simulink model "pos_8mot"  (R2021a)
settings: Solver=FixedStepDiscrete  StartTime=0.0  StopTime=inf  FixedStep=0.001  RelTol=1e-3  EnableMultiTasking=on
InitFcn:
  | load("rho_CommandCalib.mat");
  | run("importCmd.m")
model workspace (MAT data in the model file):
  positionCmd = [145.742 145.741 145.741 145.74 145.74 145.739 145.738 145.738 145.737 145.737 145.736 145.735 ... (560000 elements, 70000x8)]
  tempsTraj = [25 25 20]
values from neighbouring files (symbols this model uses):
  rho_CommandCalib = [325.033 325.033 325.033 325.033 325.033 325.033 325.033 325.033 325.033 325.033 325.033 325.033 ... (80000 elements, 10000x8)]    [rho_CommandCalib.mat]
undefined symbols (not defined in the file or in its folder): rho_CommandCircXY, rho_CommandCroixTilt, rho_CommandCroixXY, rho_CommandInclinaison, rho_CommandInclinaisonInterieure, rho_CommandPickAndPlace, rho_CommandPickAndPlaceTilt, rho_CommandPickAndPlaceVertical, rho_CommandPickAndPlaceX, rho_CommandSinusZ, rho_CommandSinusZ_decentree, rho_CommandTwist
libraries: xpcethercatlib x64, slrealtimeethercatlib x36, commutil2 x19, slrealtimeobsoletelib x7
(part 1 of 3)
settings Model: xpc_rtwmakecfg_data=_xpcethercatlib_  SimulationMode=external  OrderedModelArguments=off  Creator=The MathWorks, Inc.  LastModifiedBy=MNLER
settings SolverCC: AlgebraicLoopSolver=TrustRegion
settings DataIOCC: LimitDataPoints=on  SaveFinalState=on  SaveFormat=StructureWithTime  InspectSignalLogs=on  ReturnWorkspaceOutputs=off
settings OptimizationCC: BlockReduction=off  OptimizeBlockIOStorage=off  BufferReuse=off  GlobalBufferReuse=off  ExpressionFolding=off  ExpressionDepthLimit=2147483647  LocalBlockOutputs=off  LifeSpan=inf  OptimizeDataStoreBuffers=off  BusAssignmentInplaceUpdate=off
settings DebuggingCC: RTPrefix=none  ReadBeforeWriteMsg=DisableAll  WriteAfterWriteMsg=DisableAll  WriteAfterReadMsg=DisableAll  UnderspecifiedInitializationDetection=Classic  MergeDetectMultiDrivingBlocksExec=none  MaxConsecutiveZCsMsg=warning  SolverPrmCheckMsg=warning  InheritedTsInSrcMsg=none  MultiTaskDSMMsg=none  MultiTaskCondExecSysMsg=none  MultiTaskRateTransMsg=warning  TasksWithSamePriorityMsg=none  SigSpecEnsureSampleTimeMsg=none  Int32ToFloatConvMsg=none  ParameterDowncastMsg=none  ParameterOverflowMsg=none  ParameterPrecisionLossMsg=none  ParameterTunabilityLossMsg=none  FcnCallInpInsideContextMsg=warning  BusObjectLabelMismatch=none  RootOutportRequireBusObject=none  ModelReferenceExtraNoncontSigs=none  StateNameClashWarn=warning  NonCurrentReleaseOperatingPointMsg=warning  SFUnexpectedBacktrackingDiag=warning  SFNoUnconditionalDefaultTransitionDiag=warning  SFExecutionAtInitializationDiag=none  SFMachineParentedDataDiag=warning  ArithmeticOperatorsInVariantConditions=warning
settings HardwareCC: ProdBitPerPointer=32  ProdBitPerSizeT=32  ProdBitPerPtrDiffT=32  ProdLargestAtomicFloat=None  ProdWordSize=32  ProdLongLongMode=on  ProdHWDeviceType=Generic->32-bit x86 compatible
settings ModelReferenceCC: PropagateSignalLabelsOutOfModel=off
settings SFSimCC: SimUseLocalCustomCode=off  CustomCodeUndefinedFunction=UseInterfaceOnly
settings RTWCC: Description=Simulink Real-Time  SystemTargetFile=slrt.tlc  TLCOptions=-axPCStartupFlag=1  TemplateMakefile=slrt_default_tmf  RTWVerbose=off  RTWUseLocalCustomCode=off  RTWCompilerOptimization=on
settings CodeAppCC: StateflowObjectComments=on
settings SimulinkRealTimeCC: xPCConcurrentTasks=on
settings ConfigComp: CovMetricSettings=dw  CovSaveCumulativeToWorkspaceVar=on  CovSaveSingleToWorkspaceVar=on  CovExternalEMLEnable=off  CovSFcnEnable=off

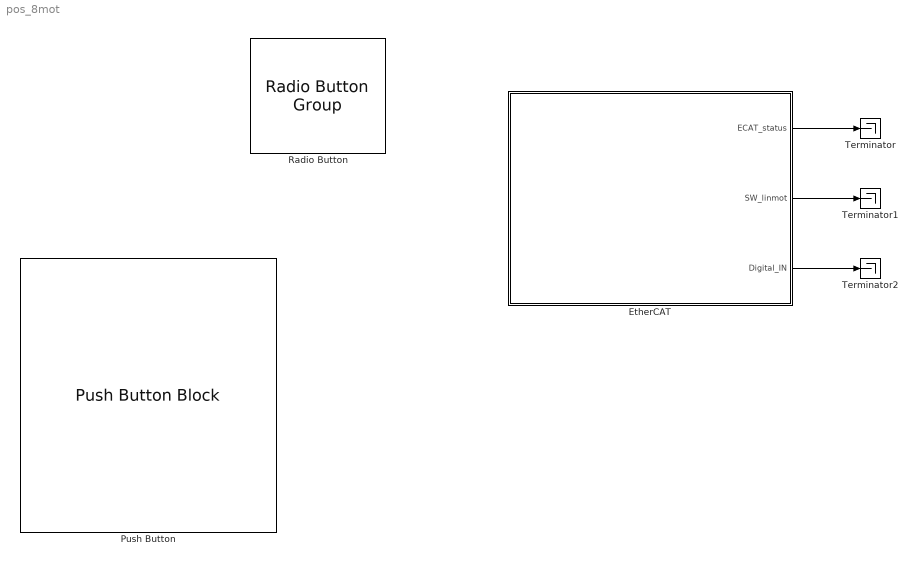
== system pos_8mot ==
  EtherCAT : Subsystem
  Push Button : PushButtonBlock  LabelPosition=Top  ButtonText=STOP!!!
  Radio Button : RadioButtonGroup  LabelPosition=Hide  SelectedLabel=Stop mode  ButtonGroupName=Mode Selection
      settings: Values={{'Stop mode', 'Homing mode', 'Position mode', 'Reset fault mode'}, [1 2 3 4]}
  Terminator : Terminator
  Terminator1 : Terminator
  Terminator2 : Terminator
  wires:
  EtherCAT/2(SW_linmot) -> Terminator1/1
  EtherCAT/1(ECAT_status) -> Terminator/1
  EtherCAT/3(Digital_IN) -> Terminator2/1
